simulink model "throttle_example"  (R2023b)
settings: Solver=FixedStepAuto  StartTime=0.0  StopTime=inf  FixedStep=0.0005  RelTol=1e-3
libraries: BeamNG_interface x1
settings Model: Creator=matti  LastModifiedBy=User
settings OptimizationCC: ReuseModelBlockBuffer=off
settings DebuggingCC: ArithmeticOperatorsInVariantConditions=warning
settings SFSimCC: CustomCodeUndefinedFunction=UseInterfaceOnly

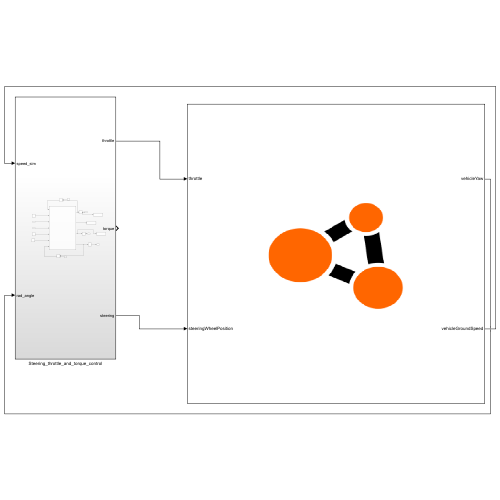
[thumbnail: Simulink's stored preview of the top-level diagram]
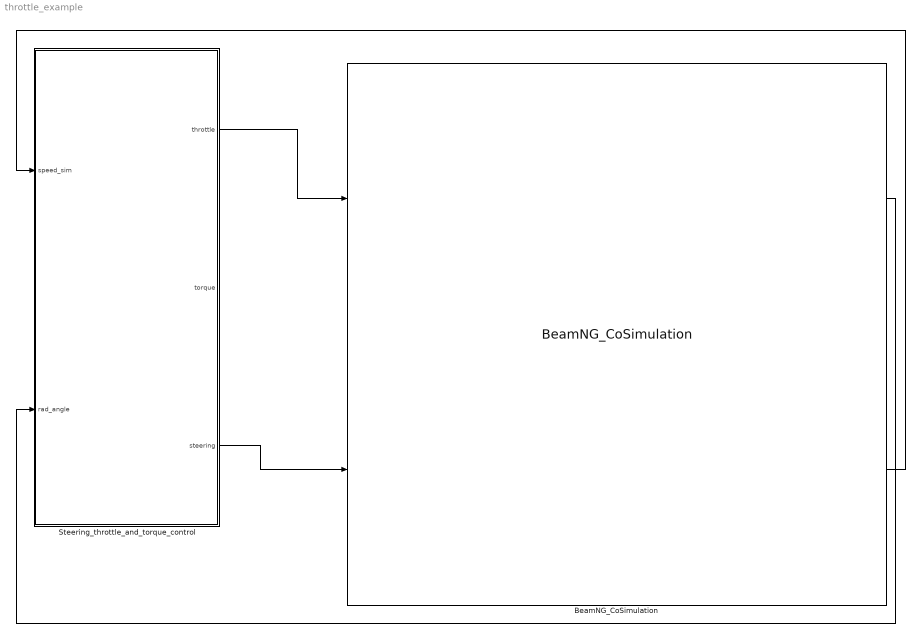
== system throttle_example ==
  BeamNG_CoSimulation : BeamNG_interface/BeamNG_CoSimulation  csvFilePath='C:\Users\User\AppData\Local\BeamNG.tech\0.32\throttle_example.csv'
  Steering_throttle_and_torque_control : Subsystem
  wires:
  Steering_throttle_and_torque_control/1(throttle) -> BeamNG_CoSimulation/1
  BeamNG_CoSimulation/2 -> Steering_throttle_and_torque_control/1(speed_sim)
  BeamNG_CoSimulation/1 -> Steering_throttle_and_torque_control/2(rad_angle)
  Steering_throttle_and_torque_control/3(steering) -> BeamNG_CoSimulation/2

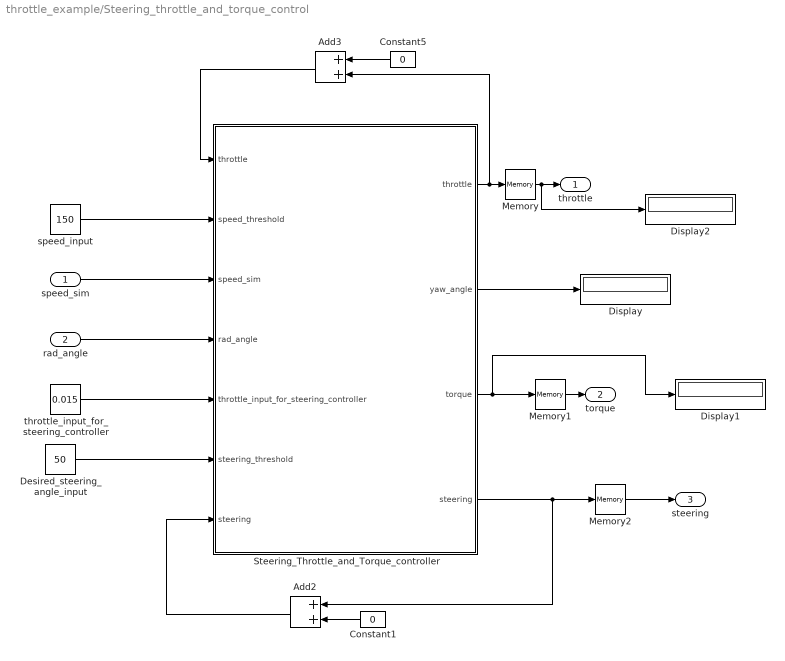
== system throttle_example/Steering_throttle_and_torque_control ==
  speed_sim : Inport
  rad_angle : Inport  Port=2
  Add2 : Sum
  Add3 : Sum
  Constant1 : Constant  Value=0
  Constant5 : Constant  Value=0
  Desired_steering_angle_input : Constant  Value=50
  Display : Display
  Display1 : Display
  Display2 : Display
  Memory : Memory
  Memory1 : Memory
  Memory2 : Memory
  Steering_Throttle_and_Torque_controller : MATLAB Function  TreatAsAtomicUnit=on
  speed_input : Constant  Value=150
  throttle_input_for_steering_controller : Constant  Value=0.015
  throttle : Outport
  torque : Outport  Port=2
  steering : Outport  Port=3
  wires:
  Memory2/1 -> steering/1
  Steering_Throttle_and_Torque_controller/3(torque) -> Memory1/1, Display1/1
  Memory1/1 -> torque/1
  Memory/1 -> throttle/1, Display2/1
  Steering_Throttle_and_Torque_controller/2(yaw_angle) -> Display/1
  throttle_input_for_steering_controller/1 -> Steering_Throttle_and_Torque_controller/5(throttle_input_for_steering_controller)
  speed_sim/1 -> Steering_Throttle_and_Torque_controller/3(speed_sim)
  rad_angle/1 -> Steering_Throttle_and_Torque_controller/4(rad_angle)
  Steering_Throttle_and_Torque_controller/4(steering) -> Add2/1, Memory2/1
  Add3/1 -> Steering_Throttle_and_Torque_controller/1("throttle ")
  Constant1/1 -> Add2/2
  Add2/1 -> Steering_Throttle_and_Torque_controller/7("steering ")
  Steering_Throttle_and_Torque_controller/1(throttle) -> Add3/2, Memory/1
  Constant5/1 -> Add3/1
  Desired_steering_angle_input/1 -> Steering_Throttle_and_Torque_controller/6(steering_threshold)
  speed_input/1 -> Steering_Throttle_and_Torque_controller/2(speed_threshold)

== matlab function throttle_example/Steering_throttle_and_torque_control/Steering_Throttle_and_Torque_controller ==
  data: throttle input; throttle output; yaw_angle output; torque output; steering output; speed_threshold input; speed_sim input; rad_angle input; throttle_input_for_steering_controller input; steering_threshold input; steering input
function [throttle,yaw_angle,torque,steering]= Controller(throttle,speed_threshold,speed_sim,rad_angle,throttle_input_for_steering_controller,steering_threshold,steering)
    % Steering 
    steering_clearance=1; % in degrees
    % here's converting the angle from radiant to degree      
    yaw_angle=rad_angle*(180/pi);
    if yaw_angle <= (steering_threshold-steering_clearance)
    steering=-throttle_input_for_steering_controller;
    end   

    if  yaw_angle > (steering_threshold)
    steering=throttle_input_for_steering_controller;
    end   


    % Throttle and Torque 
    speed_clearance=10;
    actual_speed=speed_sim*3.6;
    if actual_speed <= 5
    torque = 270 ; 
    throttle=0.5;
    elseif actual_speed <= (speed_threshold-speed_clearance)
    throttle=0.5;
    torque = 200 ; 
    elseif  actual_speed > (speed_threshold)
    throttle=-0.05;
    torque = 65; 
    else
    torque = 170; 
    end
    end
